simulink model "LeadController"  (R2018b)
settings: Solver=VariableStepAuto  StartTime=0.0  StopTime=10  RelTol=1e-3
settings Model: Creator=User  LastModifiedBy=User

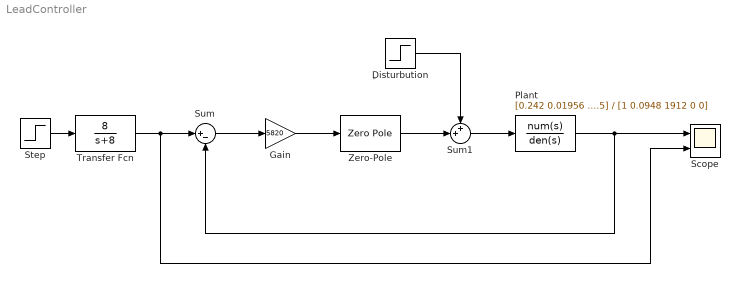
== system LeadController ==
  Gain : Gain  Gain=5820
  Plant : TransferFcn  Numerator=[0.242 0.01956 394.5]  Denominator=[1 0.0948 1912 0 0]
  Scope : Scope  NumInputPorts=2
  Step : Step  SampleTime=0
  Sum : Sum  Inputs=|+-
  Sum1 : Sum  Inputs=++|
  Transfer Fcn : TransferFcn  Numerator=[8]  Denominator=[1 8]
  Zero-Pole : ZeroPole  Zeros=[-1]  Poles=[-37.94]
  ِDisturbution : Step  SampleTime=0
  wires:
  Sum/1 -> Gain/1
  Sum1/1 -> Plant/1
  Step/1 -> Transfer Fcn/1
  Plant/1 -> Sum/2, Scope/1
  Gain/1 -> Zero-Pole/1
  Zero-Pole/1 -> Sum1/2
  ِDisturbution/1 -> Sum1/1
  Transfer Fcn/1 -> Sum/1, Scope/2
